simulink model "SuspenseSystem"  (Simulink 9.3)
settings: Solver=VariableStepAuto  StartTime=0.0  StopTime=10.0  RelTol=1e-3
values from neighbouring files (symbols this model uses):
  b = 500    [SuspenseSystemODE.m]    (also in constants1.m)
  ks = 10000    [SuspenseSystemODE.m]    (also in constants1.m)
  kw = 500000    [SuspenseSystemODE.m]    (also in constants1.m)
  m1 = 10    [SuspenseSystemODE.m]    (also in constants1.m)
  m2 = 350    [SuspenseSystemODE.m]    (also in constants1.m)
settings Model: Creator=lucanhen  LastModifiedBy=lucandh1
settings DataIOCC: SaveFormat=Dataset  SignalLoggingSaveFormat=Dataset  ReturnWorkspaceOutputs=on
settings OptimizationCC: LifeSpan=auto
settings DebuggingCC: UnderspecifiedInitializationDetection=Simplified  MergeDetectMultiDrivingBlocksExec=error  FcnCallInpInsideContextMsg=error  SFUnexpectedBacktrackingDiag=error  SFNoUnconditionalDefaultTransitionDiag=error  SFExecutionAtInitializationDiag=warning  ArithmeticOperatorsInVariantConditions=error
settings HardwareCC: ProdBitPerPointer=64  ProdBitPerSizeT=64  ProdBitPerPtrDiffT=64  ProdLargestAtomicFloat=Float  ProdIntDivRoundTo=Zero  ProdEndianess=LittleEndian  ProdWordSize=64  ProdHWDeviceType=Intel->x86-64 (Windows64)
settings ModelReferenceCC: PropagateSignalLabelsOutOfModel=on
settings SFSimCC: SimUseLocalCustomCode=on
settings RTWCC: RTWUseLocalCustomCode=on
settings CodeAppCC: StateflowObjectComments=off
settings GRTTargetCC: TargetLangStandard=C99 (ISO)  CombineOutputUpdateFcns=on  GRTInterface=off
settings ConfigComp: CovMetricSettings=dwe  CovHtmlReporting=off  CovSaveCumulativeToWorkspaceVar=off  CovSaveSingleToWorkspaceVar=off  CovExternalEMLEnable=on

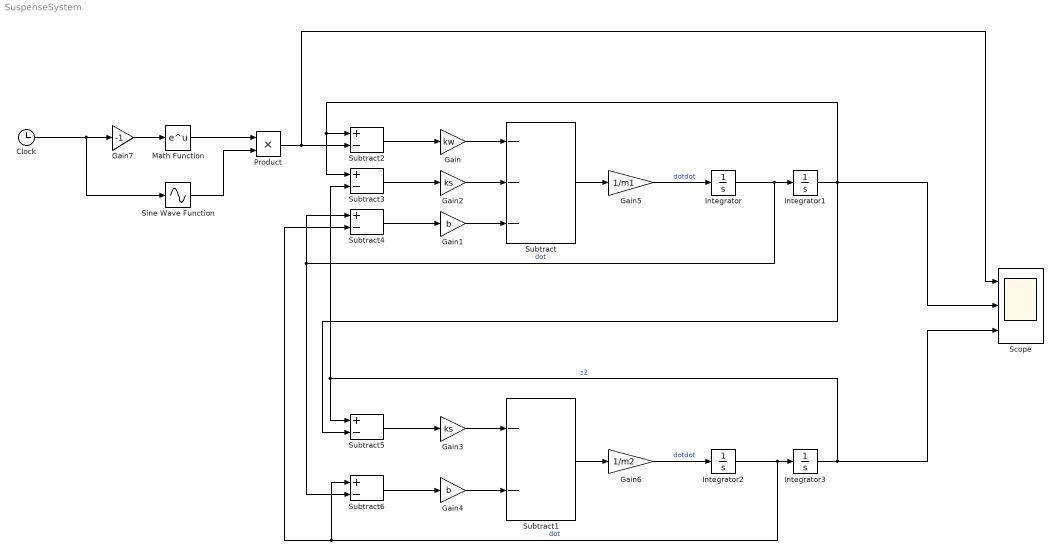
== system SuspenseSystem ==
  Clock : Clock
  Gain : Gain  Gain=kw
  Gain1 : Gain  Gain=b
  Gain2 : Gain  Gain=ks
  Gain3 : Gain  Gain=ks
  Gain4 : Gain  Gain=b
  Gain5 : Gain  Gain=1/m1
  Gain6 : Gain  Gain=1/m2
  Gain7 : Gain  Gain=-1
  Integrator{,1..3} (4 alike) : Integrator
  Math Function : Math  SaturateOnIntegerOverflow=on
  Product : Product
  Scope : Scope  NumInputPorts=3
  Sine Wave Function : Sin  TimeSource=Use external signal  SampleTime=0
  Subtract : Sum  Inputs=---
  Subtract1 : Sum  Inputs=--
  Subtract{2..6} (5 alike) : Sum  Inputs=+-
  wires:
  Gain1/1 -> Subtract/3
  Gain2/1 -> Subtract/2
  Gain/1 -> Subtract/1
  Gain3/1 -> Subtract1/1
  Gain4/1 -> Subtract1/2
  Subtract/1 -> Gain5/1
  Subtract1/1 -> Gain6/1
  Gain5/1 -> Integrator/1  "dotdot"
  Integrator/1 -> Subtract6/2, Subtract4/1, Integrator1/1  "dot"
  Integrator3/1 -> Subtract5/1, Subtract3/2, Scope/3  "z2"
  Integrator2/1 -> Subtract6/1, Subtract4/2, Integrator3/1  "dot"
  Gain6/1 -> Integrator2/1  "dotdot"
  Integrator1/1 -> Subtract5/2, Scope/2, Subtract3/1, Subtract2/1
  Subtract2/1 -> Gain/1
  Subtract3/1 -> Gain2/1
  Subtract4/1 -> Gain1/1
  Subtract6/1 -> Gain4/1
  Subtract5/1 -> Gain3/1
  Product/1 -> Subtract2/2, Scope/1
  Math Function/1 -> Product/1
  Sine Wave Function/1 -> Product/2
  Gain7/1 -> Math Function/1
  Clock/1 -> Sine Wave Function/1, Gain7/1
